simulink model "m02_linearization_model"  (R2021a)
settings: Solver=VariableStepAuto  StartTime=0.0  StopTime=10.0  RelTol=1e-3
libraries: acolibjan22 x1
settings Model: Creator=e102261  LastModifiedBy=e102261
settings SolverCC: AlgebraicLoopSolver=TrustRegion
settings DebuggingCC: ArithmeticOperatorsInVariantConditions=warning
settings SFSimCC: CustomCodeUndefinedFunction=UseInterfaceOnly

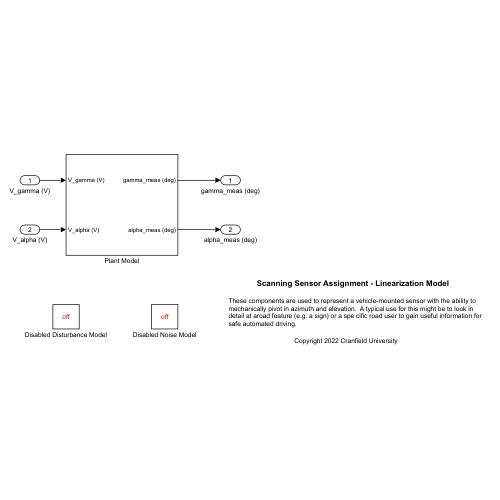
[thumbnail: Simulink's stored preview of the top-level diagram]
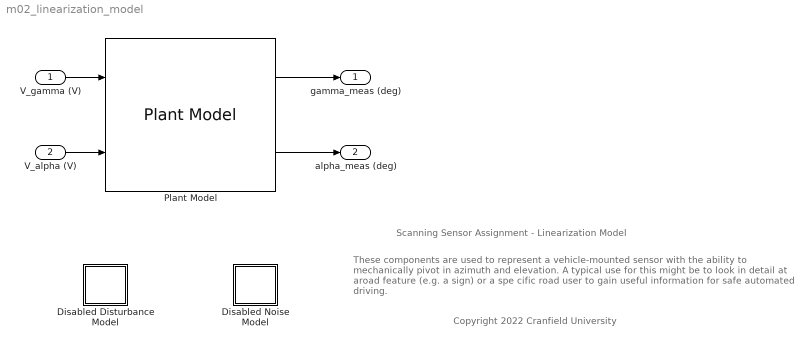
== system m02_linearization_model ==
  note: These components are used to represent a vehicle-mounted sensor with the ability to mechanically pivot in azimuth and elevation.  A typical use for this might be to look in
      | detail at aroad feature (e.g. a sign) or a spe cific road user to gain useful information for
      | safe automated driving.
  note: Scanning Sensor Assignment - Linearization Model
  note: Copyright 2022 Cranfield University
  V_gamma (V) : Inport
  V_alpha (V) : Inport  Port=2
  Disabled Disturbance Model : Subsystem
      mask Display:
      | color('red');
      | fprintf('off')
  Disabled Noise Model : Subsystem
      mask Display:
      | color('red');
      | fprintf('off')
  Plant Model : acolibjan22/Plant Model  X0=0
  gamma_meas (deg) : Outport
  alpha_meas (deg) : Outport  Port=2
  wires:
  V_gamma (V)/1 -> Plant Model/1
  V_alpha (V)/1 -> Plant Model/2
  Plant Model/1 -> gamma_meas (deg)/1
  Plant Model/2 -> alpha_meas (deg)/1

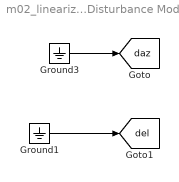
== system m02_linearization_model/Disabled Disturbance Model ==
  Ground1 : Ground
  Ground3 : Ground
  tag scope: daz=global, del=global
  wires:
  Ground3/1 -> [daz]
  Ground1/1 -> [del]

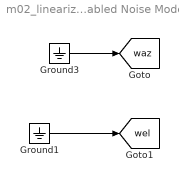
== system m02_linearization_model/Disabled Noise Model ==
  Ground1 : Ground
  Ground3 : Ground
  tag scope: waz=global, wel=global
  wires:
  Ground1/1 -> [wel]
  Ground3/1 -> [waz]
